simulink model "battSysID_EKF_age"  (R2019b)
settings: Solver=VariableStepAuto  StartTime=0.0  StopTime=tcyc(end)  RelTol=1e-3  AbsTol=1e-3  EnableMultiTasking=on
PreLoadFcn:
  | sohEstimation_ini
values from neighbouring files (symbols this model uses):
  Ts = 0.01    [sohEstimation_ini.m]
  Ts_noise = .1    (= 0.1)    [sohEstimation_ini.m]
undefined symbols (not defined in the file or in its folder): Battery
libraries: fl_lib x7, nesl_utility x5, simulink x3, sharedTrackingLibrary x1, ee_lib x1, dspstat3 x1
settings Model: Creator=jgazzarr  LastModifiedBy=jgazzarr
settings SolverCC: AutoScaleAbsTol=off
settings DataIOCC: LimitDataPoints=on  MaxDataPoints=10000  ReturnWorkspaceOutputs=off
settings OptimizationCC: DefaultParameterBehavior=Inlined  PassReuseOutputArgsAs=Individual arguments  EfficientTunableParamExpr=on
settings DebuggingCC: ParameterTunabilityLossMsg=error  AllowSymbolicDim=off  PregeneratedLibrarySubsystemCodeDiagnostic=none  SFUnexpectedBacktrackingDiag=warning  SFNoUnconditionalDefaultTransitionDiag=warning  SFExecutionAtInitializationDiag=none  ArithmeticOperatorsInVariantConditions=warning
settings HardwareCC: ProdBitPerChar=16  ProdBitPerInt=16  ProdBitPerPointer=32  ProdBitPerSizeT=32  ProdBitPerPtrDiffT=32  ProdLargestAtomicInteger=Integer  ProdLargestAtomicFloat=None  ProdWordSize=16  ProdHWDeviceType=Texas Instruments->C2000
settings SFSimCC: SimUseLocalCustomCode=off  MATLABDynamicMemAlloc=off  CustomCodeUndefinedFunction=UseInterfaceOnly
settings RTWCC: SystemTargetFile=ert.tlc  GenCodeOnly=on  TemplateMakefile=ert_default_tmf  GenerateReport=on  RTWUseLocalCustomCode=off  IncludeHyperlinkInReport=on  LaunchReport=on  GenerateTraceInfo=on  GenerateTraceReport=on  GenerateTraceReportSl=on  GenerateTraceReportSf=on  GenerateTraceReportEml=on
settings CodeAppCC: ForceParamTrailComments=on  IgnoreCustomStorageClasses=off  OperatorAnnotations=on  SimulinkDataObjDesc=on  SFDataObjDesc=on  InsertBlockDesc=on
settings ERTTargetCC: GenerateSampleERTMain=on  InlinedParameterPlacement=NonHierarchical  ERTCustomFileTemplate=example_file_process.tlc
settings ConfigComp: CovMetricSettings=dw  CovHtmlReporting=on  CovSaveCumulativeToWorkspaceVar=on  CovSaveSingleToWorkspaceVar=on  CovExternalEMLEnable=off  CovSFcnEnable=off
settings SimscapeCC: SimscapeLogType=all  SimscapeLogLimitData=off  SimscapeLogDataHistory=10000

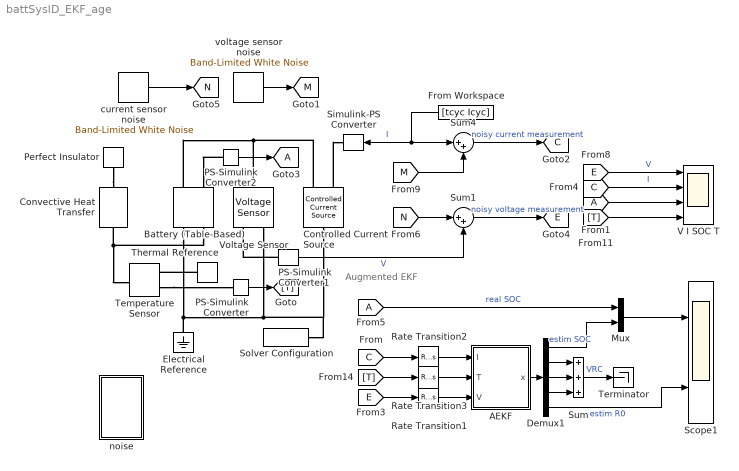
== system battSysID_EKF_age ==
  note: Augmented EKF
  AEKF : Subsystem
  Battery (Table-Based) : ee_lib/Sources/Battery (Table-Based)  SOC_vec=Battery(1).SOC_LUT  T_dependence=ee.enum.temperature_dependence.yes  T_vec=Battery(1).Temperature_LUT K  V0_mat=Battery(1).Em_LUT V  V0_vec=[3.1, 3.27, 3.31, 3.5] V  R0_mat=Battery(1).R0_LUT Ohm  R0_vec=[.015, .017, .012, .013] Ohm  AH_vec=Battery(1).Capacity_LUT hr*A  AH=4.1 hr*A  prm_leak=ee.enum.battery.prm_leak.disabled  Rleak_vec=[8000, 7000, 6000] Ohm  Rleak=7e3 Ohm  prm_dyn=ee.enum.battery.prm_dyn.rc3  R1_mat=Battery(1).R1_LUT Ohm  R1_vec=[.076, .022, .007, .043] Ohm  tau1_mat=Battery(1).t1_LUT s  tau1_vec=[148, 110, 27, 22] s  R2_mat=Battery(1).R2_LUT Ohm  R2_vec=[.382, .006, .007, .956] Ohm  tau2_mat=Battery(1).t2_LUT s  tau2_vec=[44, 24, 14, 13419] s  R3_mat=Battery(1).R3_LUT Ohm  R3_vec=[.382, .006, .007, .956] Ohm  tau3_mat=Battery(1).t3_LUT s  tau3_vec=[44, 24, 14, 13419] s  R4_mat=[.014, .382, .407; .028, .006, .007; .014, .007, .006; .333, .956, .912] Ohm  R4_vec=[.382, .006, .007, .956] Ohm  tau4_mat=[1, 44, 5644; 11, 24, 506; 2, 14, 330; 3310, 13419, 30216] s  tau4_vec=[44, 24, 14, 13419] s  R5_mat=[.014, .382, .407; .028, .006, .007; .014, .007, .006; .333, .956, .912] Ohm  R5_vec=[.382, .006, .007, .956] Ohm  tau5_mat=[1, 44, 5644; 11, 24, 506; 2, 14, 330; 3310, 13419, 30216] s  tau5_vec=[44, 24, 14, 13419] s  prm_fade=ee.enum.battery.prm_fade.equations  N0=10  dV0=0  dR0=10000/10  dAH=0  dRleak=0  dR1=0  dR2=0  dR3=0  dR4=0  dR5=0  N0vec=[100, 200, 300]  Tfadevec=[298.15, 323.15] K  dV0vec=[0, 0, 0]  dR0vec=[0, 0, 0]  dAHvec=[0, 0, 0]  dRleakvec=[0, 0, 0]  dR1vec=[0, 0, 0]  dR2vec=[0, 0, 0]  dR3vec=[0, 0, 0]  dR4vec=[0, 0, 0]  dR5vec=[0, 0, 0]  dV0mat=[0, 0; 0, 0; 0, 0]  dR0mat=[0, 0; 0, 0; 0, 0]  dAHmat=[0, 0; 0, 0; 0, 0]  dRleakmat=[0, 0; 0, 0; 0, 0]  dR1mat=[0, 0; 0, 0; 0, 0]  dR2mat=[0, 0; 0, 0; 0, 0]  dR3mat=[0, 0; 0, 0; 0, 0]  dR4mat=[0, 0; 0, 0; 0, 0]  dR5mat=[0, 0; 0, 0; 0, 0]  temperature=Battery(1).T_init K  i_specify=off  i_priority=None  i=0 A  i_nominal_specify=off  i_nominal_unit=A  i_nominal_value=1  v_specify=off  v_priority=None  v=0 V  v_nominal_specify=off  v_nominal_unit=V  v_nominal_value=1  stateOfCharge_specify=on  stateOfCharge_priority=High  stateOfCharge=Battery(1).SOC0  stateOfCharge_nominal_specify=off  stateOfCharge_nominal_unit=1  stateOfCharge_nominal_value=1  num_cycles_specify=off  num_cycles_priority=High  num_cycles=0  num_cycles_nominal_specify=off  num_cycles_nominal_unit=1  num_cycles_nominal_value=1  thermal_mass=Battery(1).cell_Cp_heat * Battery(1).cell_mass J/K  temperature_specify=on  temperature_priority=High  temperature_nominal_specify=off  temperature_nominal_unit=K  temperature_nominal_value=1
      settings: SourceProductName=Simscape Electrical  SourceProductBaseCode=PS  InternalSimscapePortConfiguration="{\"Bottom\":[],\"Left\":[{\"id\":\"p\",\"label\":\"+\",\"type\":\"foundation.electrical.electrical\"},{\"id\":\"soc\",\"label\":\"SOC\",\"type\":\"output\"}],\"Right\":[{\"id\":\"n\",\"label\":\"-\",\"type\":\"foundation.electrical.electrical\"},{\"id\":\"H\",\"label\":\"H\",\"type\":\"foundation.thermal.thermal\"}],\"Top\":[]}"
  Controlled Current Source : fl_lib/Electrical/Electrical Sources/Controlled Current Source
  Convective Heat Transfer : fl_lib/Thermal/Thermal Elements/Convective Heat Transfer  area=1e-4 m^2  heat_tr_coeff=20 W/(m^2 * K)  T_specify=off  T_priority=None  T=0 K  T_nominal_specify=off  T_nominal_unit=K  T_nominal_value=1  Q_specify=off  Q_priority=None  Q=0 W  Q_nominal_specify=off  Q_nominal_unit=W  Q_nominal_value=1
  Demux1 : Demux  Outputs=5
  Electrical Reference : fl_lib/Electrical/Electrical Elements/Electrical Reference
      settings: SourceProductName=Foundation Library
  From Workspace : FromWorkspace  VariableName=[tcyc Icyc]  SampleTime=0
  Mux : Mux  Inputs=2
  PS-Simulink Converter : nesl_utility/PS-Simulink Converter  PhysicalDomain=network_engine_domain  SubClassName=ps_output  LeftPortType=input  RightPortType=output  PseudoPeriodic=off  Frequencies=[]  Unit=inherit  AffineConversion=off
  PS-Simulink Converter1 : nesl_utility/PS-Simulink Converter  PhysicalDomain=network_engine_domain  SubClassName=ps_output  LeftPortType=input  RightPortType=output  PseudoPeriodic=off  Frequencies=[]  Unit=1  AffineConversion=off
  PS-Simulink Converter2 : nesl_utility/PS-Simulink Converter  PhysicalDomain=network_engine_domain  SubClassName=ps_output  LeftPortType=input  RightPortType=output  PseudoPeriodic=off  Frequencies=[]  Unit=inherit  AffineConversion=off
  Perfect Insulator : fl_lib/Thermal/Thermal Elements/Perfect Insulator  T_specify=off  T_priority=None  T=0 K  T_nominal_specify=off  T_nominal_unit=K  T_nominal_value=1
      settings: SourceProductName=Simscape
  Rate Transition1 : RateTransition
  Rate Transition2 : RateTransition
  Rate Transition3 : RateTransition
  Scope1 : Scope  NumInputPorts=2
  Simulink-PS Converter : nesl_utility/Simulink-PS Converter  PhysicalDomain=network_engine_domain  SubClassName=ps_input  LeftPortType=input  RightPortType=output  PseudoPeriodic=off  Frequencies=[]  NoiseDistribution=none  NoiseParameters=[]  Unit=1  AffineConversion=off  FilteringAndDerivatives=zero  SimscapeFilterOrder=1  InputFilterTimeConstant=0.001  UdotUserProvided=1
  Solver Configuration : nesl_utility/Solver Configuration  PhysicalDomain=network_engine_domain  SubClassName=solver  LeftPortType=input  RightPortType=generic  Tones=[]  Harmonics=[]  SimulateNoise=off  Profile=off  UseLocalSampling=off  EnableSwitchedLinearOptims=on  FrequencyDomain=off  UseCCode=off  RelTol=0.001  AbsTol=1e-06  MinStep=1e-09  ToWorkspace=off  RevertToSquareIcSolve=off  NumHomotopyIterations=100  PhasorMode=off  PhasorModeNumHarmonics=1  DoDC=off  ResidualTolerance=1e-09  UseLocalSolver=off  LocalSolverChoice=NE_BACKWARD_EULER_ADVANCER  LocalSolverSampleTime=0.001  DoFixedCost=off  MaxNonlinIter=3  MaxModeIter=2  LinearAlgebra=Sparse  EquationFormulation=NE_TIME_EF  DelaysMemoryBudget=1024  AutomaticFiltering=on  FilteringTimeConstant=0.001  PartitionStorageMethod=AS_NEEDED  PartitionMemoryBudget=1024  PartitionMethod=FAST
  Sum : Sum  Inputs=+++
  Sum1 : Sum  Inputs=|++
  Sum4 : Sum  Inputs=|++
  Temperature Sensor : fl_lib/Thermal/Thermal Sensors/Temperature Sensor
  Terminator : Terminator
  Thermal Reference : fl_lib/Thermal/Thermal Elements/Thermal Reference
  V I SOC T : Scope  NumInputPorts=4
  Voltage Sensor : fl_lib/Electrical/Electrical Sensors/Voltage Sensor
  current sensor noise : simulink/Sources/Band-Limited White Noise  Cov=1E-6  Ts=Ts_noise  seed=[23341]
  noise : Subsystem
  voltage sensor noise : simulink/Sources/Band-Limited White Noise  Cov=1E-6  Ts=Ts_noise  seed=[1]
  tag scope: A=global, C=global, E=global, M=global, N=global
  wires:
  From Workspace/1 -> Sum4/1, Simulink-PS Converter/1  "I"
  Demux1/1 -> Mux/2  "estim SOC"
  Mux/1 -> Scope1/1
  Sum1/1 -> [E]  "noisy voltage measurement"
  [E] -> Rate Transition1/1
  [A] -> Mux/1  "real SOC"
  current sensor noise/1 -> [N]
  Sum4/1 -> [C]  "noisy current measurement"
  [C] -> Rate Transition2/1
  PS-Simulink Converter1/1 -> Sum1/2  "V"
  [A] -> V I SOC T/3
  [C] -> V I SOC T/2  "I"
  [E] -> V I SOC T/1  "V"
  voltage sensor noise/1 -> [M]
  [N] -> Sum1/1
  [M] -> Sum4/2
  [T] -> V I SOC T/4
  Rate Transition2/1 -> AEKF/1(I)
  PS-Simulink Converter/1 -> [T]
  Rate Transition1/1 -> AEKF/3(V)
  [T] -> Rate Transition3/1
  Rate Transition3/1 -> AEKF/2(T)
  AEKF/1(x) -> Demux1/1
  PS-Simulink Converter2/1 -> [A]
  Demux1/5 -> Scope1/2  "estim R0"
  Demux1/2 -> Sum/1
  Demux1/3 -> Sum/2
  Demux1/4 -> Sum/3
  Sum/1 -> Terminator/1  "VRC"
  connections:
  Electrical Reference/LConn1 -- Battery (Table-Based)/RConn1 -- Solver Configuration/RConn1 -- Controlled Current Source/LConn1 -- Voltage Sensor/RConn2
  Battery (Table-Based)/RConn2 -- Temperature Sensor/LConn1 -- Convective Heat Transfer/LConn1
  Controlled Current Source/RConn2 -- Battery (Table-Based)/LConn1 -- Voltage Sensor/LConn1
  Perfect Insulator/LConn1 -- Convective Heat Transfer/RConn1
  Controlled Current Source/RConn1 -- Simulink-PS Converter/RConn1
  PS-Simulink Converter1/LConn1 -- Voltage Sensor/RConn1
  Temperature Sensor/RConn2 -- PS-Simulink Converter/LConn1
  PS-Simulink Converter2/LConn1 -- Battery (Table-Based)/LConn2
  Thermal Reference/LConn1 -- Temperature Sensor/RConn1

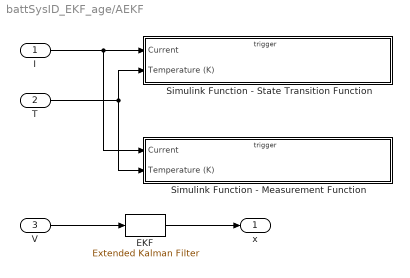
== system battSysID_EKF_age/AEKF ==
  I : Inport
  T : Inport  Port=2
  V : Inport  Port=3
  EKF : sharedTrackingLibrary/Extended Kalman Filter  StateTransitionFcn=batteryStateFcn  HasStateTransitionJacobianFcn=off  HasAdditiveProcessNoise=Additive  ProcessNoise=diag([1e-3 1 1 1 1e-2]*1e-5)  HasTimeVaryingProcessNoise=off  HasStateTransitionFcnExtraArgument=0  InitialState=[0.6 0 0 0 0.01]  InitialStateCovariance=[1e8 1 1 1 1e4]*1e-5  MeasurementFcn1=batteryMeasurementFcn  HasMeasurementJacobianFcn1=off  HasMeasurementEnablePort1=off  HasAdditiveMeasurementNoise1=Additive  MeasurementNoise1=1e-6 + 7.9  HasTimeVaryingMeasurementNoise1=off  HasMeasurementFcnExtraArgument1=0  MeasurementFcn2=myMeasurementFcn  HasMeasurementJacobianFcn2=off  HasMeasurementEnablePort2=off  HasAdditiveMeasurementNoise2=Additive  MeasurementNoise2=1  HasTimeVaryingMeasurementNoise2=off  HasMeasurementFcnExtraArgument2=0  MeasurementFcn3=myMeasurementFcn  HasMeasurementJacobianFcn3=off  HasMeasurementEnablePort3=off  HasAdditiveMeasurementNoise3=Additive  MeasurementNoise3=1  HasTimeVaryingMeasurementNoise3=off  HasMeasurementFcnExtraArgument3=0  MeasurementFcn4=myMeasurementFcn  HasMeasurementJacobianFcn4=off  HasMeasurementEnablePort4=off  HasAdditiveMeasurementNoise4=Additive  MeasurementNoise4=1  HasTimeVaryingMeasurementNoise4=off  HasMeasurementFcnExtraArgument4=0  MeasurementFcn5=myMeasurementFcn  HasMeasurementJacobianFcn5=off  HasMeasurementEnablePort5=off  HasAdditiveMeasurementNoise5=Additive  MeasurementNoise5=1  HasTimeVaryingMeasurementNoise5=off  HasMeasurementFcnExtraArgument5=0  EnableMultirate=off  StateTransitionFcnSampleTime=1  MeasurementFcn1SampleTime=1  MeasurementFcn2SampleTime=1  MeasurementFcn3SampleTime=1  MeasurementFcn4SampleTime=1  MeasurementFcn5SampleTime=1  UseCurrentEstimator=on  OutputStateCovariance=off  DataType=double  SampleTime=Ts  NumberOfMeasurements=1
      settings: SourceProductName=The database C:\Users\aozdemir\AppData\Roaming\MathWorks\MATLAB\R2017b\slblocks_master.db is locked, or a table in the database is locked. (database is locked)
  Simulink Function - Measurement Function : Subsystem  TreatAsAtomicUnit=on
  Simulink Function - State Transition Function : Subsystem  TreatAsAtomicUnit=on
  x : Outport  VectorParamsAs1DForOutWhenUnconnected=off
  wires:
  EKF/1 -> x/1
  I/1 -> Simulink Function - State Transition Function/1(Current), Simulink Function - Measurement Function/1(Current)
  V/1 -> EKF/1
  T/1 -> Simulink Function - State Transition Function/2(Temperature (K)), Simulink Function - Measurement Function/2(Temperature (K))

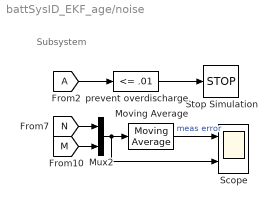
== system battSysID_EKF_age/noise ==
  note: Subsystem
  Moving Average : dspstat3/Moving Average  Method=Sliding window  ForgettingFactorPort=off  SpecifyWindowLength=on  WindowLength=100  ForgettingFactor=0.9  SimulateUsing=Code generation
  Mux2 : Mux  Inputs=2
  Scope : Scope  NumInputPorts=2
  Stop Simulation : Stop
  prevent overdischarge : simulink/Logic and Bit Operations/Compare To Constant  relop=<=  const=.01  OutDataTypeStr=boolean
  wires:
  Moving Average/1 -> Scope/1  "meas error"
  [N] -> Mux2/1
  prevent overdischarge/1 -> Stop Simulation/1
  Mux2/1 -> Scope/2, Moving Average/1
  [M] -> Mux2/2
  [A] -> prevent overdischarge/1

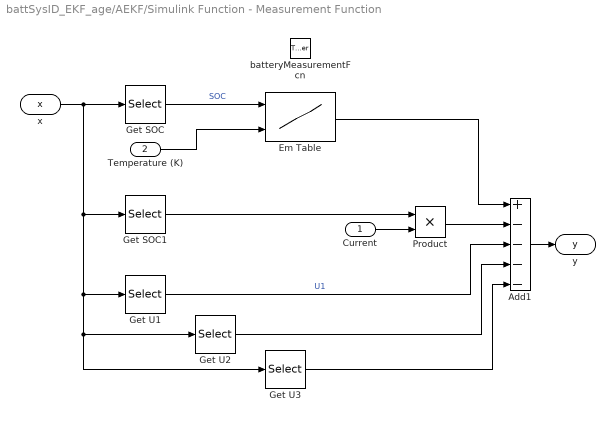
== system battSysID_EKF_age/AEKF/Simulink Function - Measurement Function ==
  Current : Inport
  Temperature (K) : Inport  Port=2
  batteryMeasurementFcn : TriggerPort  TriggerType=function-call  IsSimulinkFunction=on  FunctionName=batteryMeasurementFcn  VariantControl=Variant
  Add1 : Sum  Inputs=+----
  Em Table : Lookup_n-D  BreakpointsForDimension1=Battery.SOC_LUT  BreakpointsForDimension2=Battery.Temperature_LUT  Table=Battery.Em_LUT  InternalRulePriority=Speed  RndMeth=Simplest  InputSameDT=on
  Get SOC : Selector  InputPortWidth=5  IndexOptions=Index vector (dialog)  Indices=[1]  OutputSizes=1
  Get SOC1 : Selector  InputPortWidth=5  IndexOptions=Index vector (dialog)  Indices=[5]  OutputSizes=1
  Get U1 : Selector  InputPortWidth=5  IndexOptions=Index vector (dialog)  Indices=2  OutputSizes=1
  Get U2 : Selector  InputPortWidth=5  IndexOptions=Index vector (dialog)  Indices=3  OutputSizes=1
  Get U3 : Selector  InputPortWidth=5  IndexOptions=Index vector (dialog)  Indices=4  OutputSizes=1
  Product : Product
  x : ArgIn  DisableCoverage=on  PortDimensions=5  ArgumentName=x
  y : ArgOut  DisableCoverage=on  ArgumentName=y
  wires:
  Get U3/1 -> Add1/5
  Get U2/1 -> Add1/4
  Get U1/1 -> Add1/3  "U1"
  Product/1 -> Add1/2
  Current/1 -> Product/2
  Get SOC1/1 -> Product/1
  Temperature (K)/1 -> Em Table/2
  Add1/1 -> y/1
  Em Table/1 -> Add1/1
  Get SOC/1 -> Em Table/1  "SOC"
  x/1 -> Get SOC/1, Get SOC1/1, Get U1/1, Get U2/1, Get U3/1

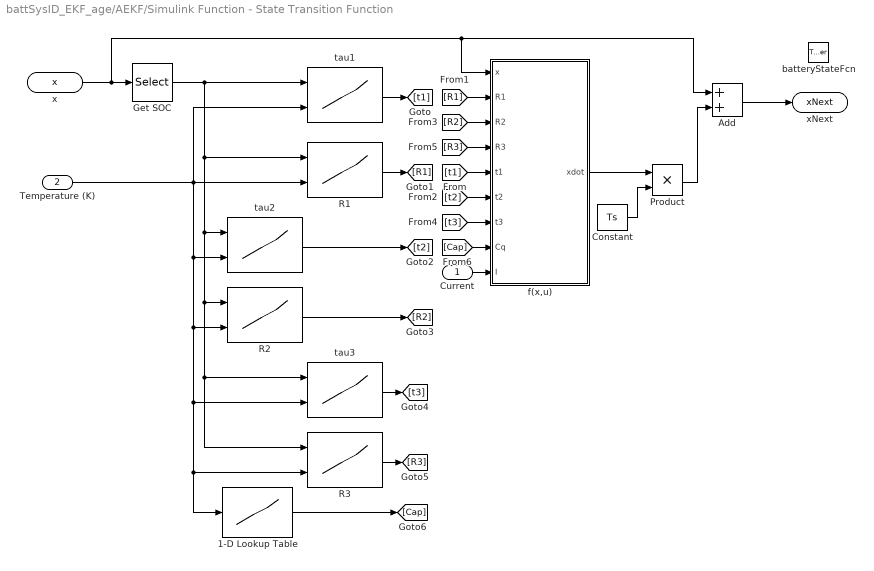
== system battSysID_EKF_age/AEKF/Simulink Function - State Transition Function ==
  Current : Inport
  Temperature (K) : Inport  Port=2
  batteryStateFcn : TriggerPort  TriggerType=function-call  IsSimulinkFunction=on  FunctionName=batteryStateFcn  VariantControl=Variant
  1-D Lookup Table : Lookup_n-D  NumberOfTableDimensions=1  BreakpointsForDimension1=Battery.Temperature_LUT  Table=Battery.Capacity_LUT  InternalRulePriority=Speed  RndMeth=Simplest  InputSameDT=on
  Add : Sum
  Constant : Constant  Value=Ts
  Get SOC : Selector  InputPortWidth=5  IndexOptions=Index vector (dialog)  Indices=1  OutputSizes=1
  Product : Product
  R1 : Lookup_n-D  BreakpointsForDimension1=Battery.SOC_LUT  BreakpointsForDimension2=Battery.Temperature_LUT  Table=Battery.R1_LUT  InternalRulePriority=Speed  RndMeth=Simplest  InputSameDT=on
  R2 : Lookup_n-D  BreakpointsForDimension1=Battery.SOC_LUT  BreakpointsForDimension2=Battery.Temperature_LUT  Table=Battery.R2_LUT  InternalRulePriority=Speed  RndMeth=Simplest  InputSameDT=on
  R3 : Lookup_n-D  BreakpointsForDimension1=Battery.SOC_LUT  BreakpointsForDimension2=Battery.Temperature_LUT  Table=Battery.R3_LUT  InternalRulePriority=Speed  RndMeth=Simplest  InputSameDT=on
  f(x,u) : MATLAB Function  TreatAsAtomicUnit=on
  tau1 : Lookup_n-D  BreakpointsForDimension1=Battery.SOC_LUT  BreakpointsForDimension2=Battery.Temperature_LUT  Table=Battery.t1_LUT  InternalRulePriority=Speed  RndMeth=Simplest  InputSameDT=on
  tau2 : Lookup_n-D  BreakpointsForDimension1=Battery.SOC_LUT  BreakpointsForDimension2=Battery.Temperature_LUT  Table=Battery.t2_LUT  InternalRulePriority=Speed  RndMeth=Simplest  InputSameDT=on
  tau3 : Lookup_n-D  BreakpointsForDimension1=Battery.SOC_LUT  BreakpointsForDimension2=Battery.Temperature_LUT  Table=Battery.t3_LUT  InternalRulePriority=Speed  RndMeth=Simplest  InputSameDT=on
  x : ArgIn  DisableCoverage=on  PortDimensions=5  ArgumentName=x
  xNext : ArgOut  DisableCoverage=on  PortDimensions=5  ArgumentName=xNext
  wires:
  tau1/1 -> [t1]
  R1/1 -> [R1]
  Product/1 -> Add/2
  f(x,u)/1(xdot) -> Product/1
  Constant/1 -> Product/2
  Current/1 -> f(x,u)/9(I)
  Get SOC/1 -> tau1/1, tau2/1, R2/1, tau3/1, R3/1, R1/1
  Temperature (K)/1 -> tau1/2, R1/2, tau2/2, R2/2, tau3/2, R3/2, 1-D Lookup Table/1
  Add/1 -> xNext/1
  x/1 -> Get SOC/1, Add/1, f(x,u)/1(x)
  [t1] -> f(x,u)/5(t1)
  [R1] -> f(x,u)/2(R1)
  [t2] -> f(x,u)/6(t2)
  tau2/1 -> [t2]
  R2/1 -> [R2]
  [R2] -> f(x,u)/3(R2)
  tau3/1 -> [t3]
  [t3] -> f(x,u)/7(t3)
  R3/1 -> [R3]
  [R3] -> f(x,u)/4(R3)
  1-D Lookup Table/1 -> [Cap]
  [Cap] -> f(x,u)/8(Cq)

== matlab function battSysID_EKF_age/AEKF/Simulink Function - State Transition Function/f(x,u) ==
  data: x input; R1 input; R2 input; R3 input; t1 input; t2 input; t3 input; Cq input; I input; xdot output
function xdot = fx(x,R1,R2,R3,t1,t2,t3,Cq,I)
xdot = zeros(size(x));
U1 = x(2);
U2 = x(3);
U3 = x(4);
xdot(1) = -I/(3600*Cq);
xdot(2) = -1/t1*U1 + I/(t1/R1);
xdot(3) = -1/t2*U2 + I/(t2/R2);
xdot(4) = -1/t3*U3 + I/(t3/R3);
xdot(5) = 0; 

% x1 = SOC
% x2, x3, x4 = U1, U2, U3
% x5 = R0
